simulink model "Controllers_in_simulink"  (R2018a)
settings: Solver=VariableStepAuto  StartTime=0.0  StopTime=10.0  RelTol=1e-3
values from neighbouring files (symbols this model uses):
  Kp_pan = 40.5    [Controller_values.m]
  Kp_tilt = 41.1    [Controller_values.m]
  Td_pan = 0.175    [Controller_values.m]
  Td_tilt = 0.0877    [Controller_values.m]
  Ti_pan = 0.438    [Controller_values.m]
  Ti_tilt = 0.278    [Controller_values.m]
  Ts = 0.01    [Controller_values.m]
undefined symbols (not defined in the file or in its folder): DiscIntNeverNeededParam
libraries: simulink x4
settings Model: Creator=Jakob  LastModifiedBy=Jakob
settings SolverCC: ZeroCrossAlgorithm=Adaptive  AlgebraicLoopSolver=LineSearch
settings DebuggingCC: MaxConsecutiveZCsMsg=none

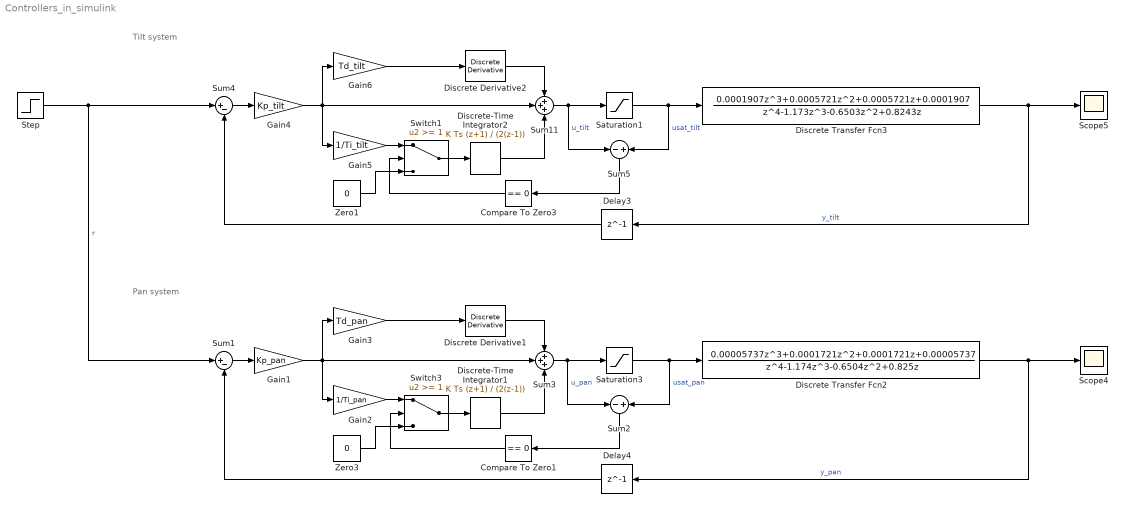
== system Controllers_in_simulink ==
  note: Pan system
  note: Tilt system
  Compare To Zero1 : simulink/Logic and Bit Operations/Compare To Zero  relop===  OutDataTypeStr=boolean
  Compare To Zero3 : simulink/Logic and Bit Operations/Compare To Zero  relop===  OutDataTypeStr=boolean
  Delay3 : Delay  DelayLength=1  SampleTime=Ts
  Delay4 : Delay  DelayLength=1  SampleTime=Ts
  Discrete Transfer Fcn2 : DiscreteTransferFcn  Numerator=[0.00005737 0.0001721 0.0001721 0.00005737]  Denominator=[1 -1.174 -0.6504 0.825 0]  SampleTime=Ts
  Discrete Transfer Fcn3 : DiscreteTransferFcn  Numerator=[0.0001907 0.0005721 0.0005721 0.0001907]  Denominator=[1 -1.173 -0.6503 0.8243 0]  SampleTime=Ts
  Discrete Derivative1 : simulink/Discrete/Discrete Derivative  gainval=1.0  ICPrevScaledInput=0.0  OutMin=[]  OutMax=[]  OutDataType=fixdt(1, 16)  OutScaling=2^-10  DoSatur=off
  Discrete Derivative2 : simulink/Discrete/Discrete Derivative  gainval=1.0  ICPrevScaledInput=0.0  OutMin=[]  OutMax=[]  OutDataType=fixdt(1, 16)  OutScaling=2^-10  DoSatur=off
  Discrete-Time Integrator1 : DiscreteIntegrator  IntegratorMethod=Integration: Trapezoidal  SampleTime=Ts  ICPrevOutput=DiscIntNeverNeededParam  ICPrevScaledInput=DiscIntNeverNeededParam
  Discrete-Time Integrator2 : DiscreteIntegrator  IntegratorMethod=Integration: Trapezoidal  SampleTime=Ts  ICPrevOutput=DiscIntNeverNeededParam  ICPrevScaledInput=DiscIntNeverNeededParam
  Gain1 : Gain  Gain=Kp_pan
  Gain2 : Gain  Gain=1/Ti_pan
  Gain3 : Gain  Gain=Td_pan
  Gain4 : Gain  Gain=Kp_tilt
  Gain5 : Gain  Gain=1/Ti_tilt
  Gain6 : Gain  Gain=Td_tilt
  Saturation1 : Saturate  UpperLimit=6  LowerLimit=-6
  Saturation3 : Saturate  UpperLimit=6  LowerLimit=-6
  Scope4 : Scope
  Scope5 : Scope
  Step : Step  Time=0  SampleTime=0
  Sum1 : Sum  Inputs=|+-
  Sum11 : Sum  Inputs=+++
  Sum2 : Sum  Inputs=-|+
  Sum3 : Sum  Inputs=+++
  Sum4 : Sum  Inputs=|+-
  Sum5 : Sum  Inputs=-|+
  Switch1 : Switch  Threshold=1
  Switch3 : Switch  Threshold=1
  Zero1 : Constant  Value=0
  Zero3 : Constant  Value=0
  wires:
  Sum1/1 -> Gain1/1
  Discrete Transfer Fcn2/1 -> Delay4/1, Scope4/1  "y_pan"
  Delay4/1 -> Sum1/2
  Discrete-Time Integrator1/1 -> Sum3/3
  Gain3/1 -> Discrete Derivative1/1
  Switch3/1 -> Discrete-Time Integrator1/1
  Sum3/1 -> Sum2/1, Saturation3/1  "u_pan"
  Gain2/1 -> Switch3/1
  Sum2/1 -> Compare To Zero1/1
  Zero3/1 -> Switch3/3
  Compare To Zero1/1 -> Switch3/2
  Gain1/1 -> Sum3/2, Gain3/1, Gain2/1
  Saturation3/1 -> Discrete Transfer Fcn2/1, Sum2/2  "usat_pan"
  Sum4/1 -> Gain4/1
  Compare To Zero3/1 -> Switch1/2
  Saturation1/1 -> Discrete Transfer Fcn3/1, Sum5/2  "usat_tilt"
  Gain4/1 -> Sum11/2, Gain6/1, Gain5/1
  Gain5/1 -> Switch1/1
  Sum11/1 -> Sum5/1, Saturation1/1  "u_tilt"
  Sum5/1 -> Compare To Zero3/1
  Zero1/1 -> Switch1/3
  Step/1 -> Sum1/1, Sum4/1  "r"
  Switch1/1 -> Discrete-Time Integrator2/1
  Gain6/1 -> Discrete Derivative2/1
  Discrete Transfer Fcn3/1 -> Delay3/1, Scope5/1  "y_tilt"
  Discrete-Time Integrator2/1 -> Sum11/3
  Delay3/1 -> Sum4/2
  Discrete Derivative2/1 -> Sum11/1
  Discrete Derivative1/1 -> Sum3/1
